simulink model "Alternanza_R_C"  (R2012b)
settings: Solver=ode45  StartTime=0.0  StopTime=10.0  RelTol=1e-3
undefined symbols (not defined in the file or in its folder): C_1, C_2, C_3, G_1, G_2, G_3, I_b_t, Q_3_0, Q_6_0, Q_9_0, V_a_t
settings Model: Creator=Roberto  LastModifiedBy=Roberto

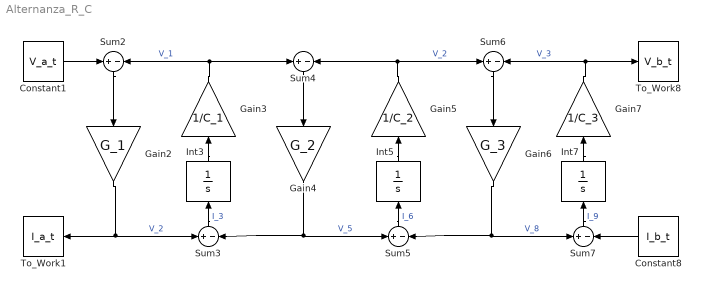
== system Alternanza_R_C ==
  Constant1 : Constant  Value=V_a_t
  Constant8 : Constant  Value=I_b_t
  Gain2 : Gain  Gain=G_1  SaturateOnIntegerOverflow=on  OutDataTypeStr=Inherit: Same as input  ParamDataTypeStr=Inherit: Same as input
  Gain3 : Gain  Gain=1/C_1  SaturateOnIntegerOverflow=on  OutDataTypeStr=Inherit: Same as input  ParamDataTypeStr=Inherit: Same as input
  Gain4 : Gain  Gain=G_2  SaturateOnIntegerOverflow=on  OutDataTypeStr=Inherit: Same as input  ParamDataTypeStr=Inherit: Same as input
  Gain5 : Gain  Gain=1/C_2  SaturateOnIntegerOverflow=on  OutDataTypeStr=Inherit: Same as input  ParamDataTypeStr=Inherit: Same as input
  Gain6 : Gain  Gain=G_3  SaturateOnIntegerOverflow=on  OutDataTypeStr=Inherit: Same as input  ParamDataTypeStr=Inherit: Same as input
  Gain7 : Gain  Gain=1/C_3  SaturateOnIntegerOverflow=on  OutDataTypeStr=Inherit: Same as input  ParamDataTypeStr=Inherit: Same as input
  Int3 : Integrator  InitialCondition=Q_3_0
  Int5 : Integrator  InitialCondition=Q_6_0
  Int7 : Integrator  InitialCondition=Q_9_0
  Sum{2..7} (6 alike) : Sum  Inputs=+|-  SaturateOnIntegerOverflow=on  InputSameDT=on  OutDataTypeStr=Inherit: Same as first input
  To_Work1 : ToWorkspace  VariableName=I_a_t
      settings: MaxDataPoints=10000
  To_Work8 : ToWorkspace  VariableName=V_b_t
      settings: MaxDataPoints=10000
  wires:
  Constant1/1 -> Sum2/1
  Gain3/1 -> Sum2/2, Sum4/1  "V_1"
  Gain2/1 -> To_Work1/1, Sum3/1  "V_2"
  Sum2/1 -> Gain2/1
  Gain4/1 -> Sum3/2, Sum5/1  "V_5"
  Sum3/1 -> Int3/1  "I_3"
  Int3/1 -> Gain3/1
  Gain5/1 -> Sum4/2, Sum6/1  "V_2"
  Sum4/1 -> Gain4/1
  Gain6/1 -> Sum5/2, Sum7/1  "V_8"
  Sum5/1 -> Int5/1  "I_6"
  Int5/1 -> Gain5/1
  Gain7/1 -> Sum6/2, To_Work8/1  "V_3"
  Sum6/1 -> Gain6/1
  Constant8/1 -> Sum7/2
  Sum7/1 -> Int7/1  "I_9"
  Int7/1 -> Gain7/1
